simulink model "simulinkStepResponse"  (R2020b)
settings: Solver=VariableStepAuto  StartTime=0.0  StopTime=10.0  RelTol=1e-3
settings Model: Creator=jaagt  LastModifiedBy=jaagt

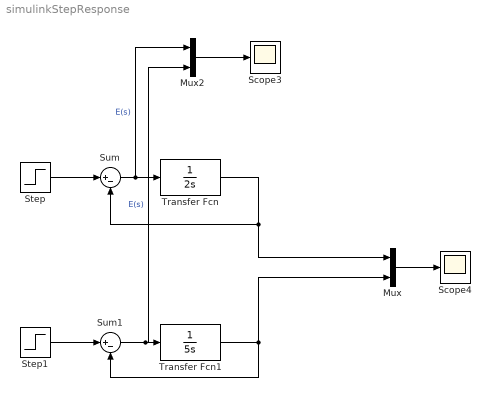
== system simulinkStepResponse ==
  Mux : Mux  Inputs=3
  Mux2 : Mux  Inputs=3
  Scope3 : Scope
  Scope4 : Scope
  Step : Step  Time=0  SampleTime=0
  Step1 : Step  Time=0  SampleTime=0
  Sum : Sum  Inputs=|+-
  Sum1 : Sum  Inputs=|+-
  Transfer Fcn : TransferFcn  Numerator=[0 1]  Denominator=[2 0]
  Transfer Fcn1 : TransferFcn  Numerator=[0 1]  Denominator=[5 0]
  wires:
  Step/1 -> Sum/1
  Sum/1 -> Mux2/1, Transfer Fcn/1  "E(s)"
  Transfer Fcn/1 -> Mux/1, Sum/2
  Sum1/1 -> Mux2/3, Transfer Fcn1/1  "E(s)"
  Transfer Fcn1/1 -> Mux/3, Sum1/2
  Step1/1 -> Sum1/1
  Mux/1 -> Scope4/1
  Mux2/1 -> Scope3/1
